simulink model "DynamicModel"  (R2021a)
settings: Solver=VariableStepAuto  StartTime=0.0  StopTime=10.0  RelTol=1e-3
libraries: pid_lib x2, simulink x1
settings Model: Creator=admin  LastModifiedBy=admin

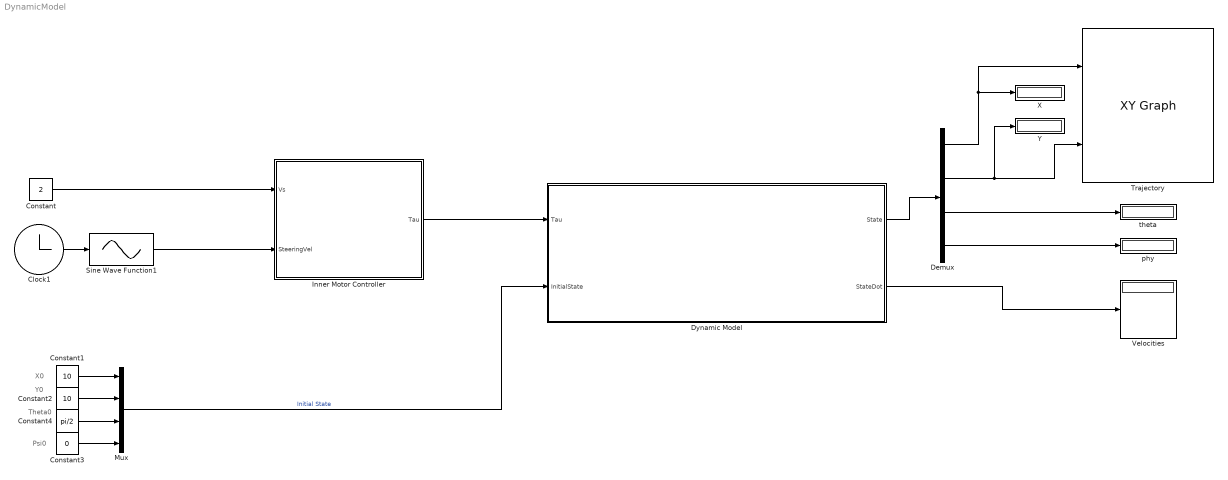
== system DynamicModel ==
  note: Y0
  note: X0
  note: Theta0
  note: Psi0
  Clock1 : Clock
  Constant : Constant  Value=2
  Constant1 : Constant  Value=10  SampleTime=0.001
  Constant2 : Constant  Value=10  SampleTime=0.001
  Constant3 : Constant  Value=0  SampleTime=0.001
  Constant4 : Constant  Value=pi/2  SampleTime=0.001
  Demux : Demux
  Dynamic Model : Subsystem
  Inner Motor Controller : Subsystem
  Mux : Mux
  Sine Wave Function1 : Sin  TimeSource=Use external signal  Amplitude=pi/4  Frequency=pi/2  SampleTime=0
  Trajectory : simulink/Sinks/XY Graph  xmin=-30  xmax=30  ymin=-30  ymax=30  st=0.001
  Velocities : Display
  X : Display
  Y : Display
  phy : Display
  theta : Display
  wires:
  Constant1/1 -> Mux/1
  Constant2/1 -> Mux/2
  Demux/3 -> theta/1
  Clock1/1 -> Sine Wave Function1/1
  Demux/2 -> Y/1, Trajectory/2
  Constant/1 -> Inner Motor Controller/1(Vs)
  Sine Wave Function1/1 -> Inner Motor Controller/2(SteeringVel)
  Constant4/1 -> Mux/3
  Demux/4 -> phy/1
  Demux/1 -> X/1, Trajectory/1
  Constant3/1 -> Mux/4
  Mux/1 -> Dynamic Model/2(InitialState)  "Initial State"
  Dynamic Model/2(StateDot) -> Velocities/1
  Dynamic Model/1(State) -> Demux/1
  Inner Motor Controller/1(Tau) -> Dynamic Model/1(Tau)

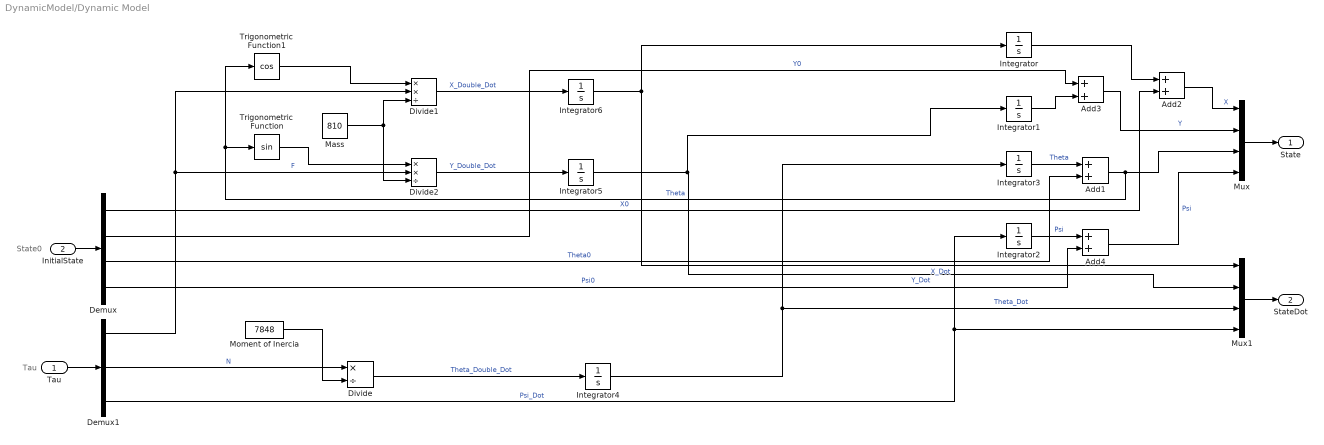
== system DynamicModel/Dynamic Model ==
  note: Tau
  note: State0
  Tau : Inport
  InitialState : Inport  Port=2
  Add{1..4} (4 alike) : Sum
  Demux : Demux
  Demux1 : Demux  Outputs=3
  Divide : Product  Inputs=*/
  Divide1 : Product  Inputs=**/
  Divide2 : Product  Inputs=**/
  Integrator{,1..6} (7 alike) : Integrator
  Mass : Constant  Value=810
  Moment of Inercia : Constant  Value=7848
  Mux : Mux
  Mux1 : Mux
  Trigonometric Function : Trigonometry
  Trigonometric Function1 : Trigonometry  Operator=cos
  State : Outport
  StateDot : Outport  Port=2
  wires:
  Mux/1 -> State/1
  Mux1/1 -> StateDot/1
  Demux1/3 -> Integrator2/1, Mux1/4  "Psi_Dot"
  Add4/1 -> Mux/4  "Psi"
  Add1/1 -> Trigonometric Function/1, Trigonometric Function1/1, Mux/3  "Theta"
  Integrator/1 -> Add2/1
  InitialState/1 -> Demux/1
  Add2/1 -> Mux/1  "X"
  Integrator1/1 -> Add3/2
  Add3/1 -> Mux/2  "Y"
  Tau/1 -> Demux1/1
  Demux/2 -> Add3/1  "Y0"
  Demux/1 -> Add2/2  "X0"
  Integrator3/1 -> Add1/1  "Theta"
  Demux/3 -> Add1/2  "Theta0"
  Integrator2/1 -> Add4/1  "Psi"
  Demux/4 -> Add4/2  "Psi0"
  Moment of Inercia/1 -> Divide/2
  Divide/1 -> Integrator4/1  "Theta_Double_Dot"
  Integrator4/1 -> Integrator3/1, Mux1/3  "Theta_Dot"
  Divide1/1 -> Integrator6/1  "X_Double_Dot"
  Divide2/1 -> Integrator5/1  "Y_Double_Dot"
  Demux1/2 -> Divide/1  "N"
  Trigonometric Function1/1 -> Divide1/1
  Trigonometric Function/1 -> Divide2/1
  Mass/1 -> Divide2/3, Divide1/3
  Demux1/1 -> Divide2/2, Divide1/2  "F"
  Integrator5/1 -> Integrator1/1, Mux1/2  "Y_Dot"
  Integrator6/1 -> Integrator/1, Mux1/1  "X_Dot"

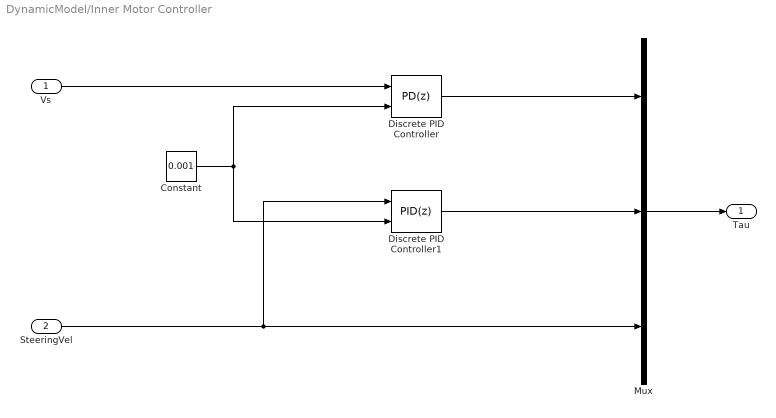
== system DynamicModel/Inner Motor Controller ==
  Vs : Inport
  SteeringVel : Inport  Port=2
  Constant : Constant  Value=0.001
  Discrete PID Controller : pid_lib/PID Controller  Controller=PD  Form=Parallel  TimeDomain=Discrete-time  UseExternalTs=on  SampleTime=-1  IntegratorMethod=Forward Euler  FilterMethod=Forward Euler  ControllerParametersSource=internal  P=1  I=1  D=0  UseFilter=on  N=100  TunerSelectOption=Transfer Function Based (PID Tuner App)  InitialConditionSource=internal  InitialConditionForIntegrator=0  InitialConditionForFilter=0  DifferentiatorICPrevScaledInput=0  ExternalReset=none  TrackingMode=off  Kt=1  LimitOutput=off  SatLimitsSource=internal  UpperSaturationLimit=inf  LowerSaturationLimit=-inf  LinearizeAsGain=off  AntiWindupMode=none  Kb=1  POutMin=[]  POutMax=[]  IOutMin=[]  IOutMax=[]  DOutMin=[]  DOutMax=[]  NOutMin=[]  NOutMax=[]  SumOutMin=[]  SumOutMax=[]  SaturationOutMin=[]  SaturationOutMax=[]  PParamMin=[]  PParamMax=[]  IParamMin=[]  IParamMax=[]  DParamMin=[]  DParamMax=[]  NParamMin=[]  NParamMax=[]  KbParamMin=[]  KbParamMax=[]  KtParamMin=[]  KtParamMax=[]  KbOutMin=[]  KbOutMax=[]  KtOutMin=[]  KtOutMax=[]  IntegratorOutMin=[]  IntegratorOutMax=[]  FilterOutMin=[]  FilterOutMax=[]  SumI1OutMin=[]  SumI1OutMax=[]  SumI2OutMin=[]  SumI2OutMax=[]  SumI3OutMin=[]  SumI3OutMax=[]  SumI4OutMin=[]  SumI4OutMax=[]  SumDOutMin=[]  SumDOutMax=[]  DifferentiatorOutMin=[]  DifferentiatorOutMax=[]  FilterDiffOutCoefMin=[]  FilterDiffOutCoefMax=[]  ReciprocalOutMin=[]  ReciprocalOutMax=[]  SumDenOutMin=[]  SumDenOutMax=[]  SumNumOutMin=[]  SumNumOutMax=[]  DivideOutMin=[]  DivideOutMax=[]  UdiffTsProdOutMin=[]  UdiffTsProdOutMax=[]  NTsProdOutMin=[]  NTsProdOutMax=[]  UintegralTsProdOutMin=[]  UintegralTsProdOutMax=[]  UngainTsProdOutMin=[]  UngainTsProdOutMax=[]  IntegratorContinuousStateAttributes=''  IntegratorStateMustResolveToSignalObject=off  IntegratorRTWStateStorageClass=Auto  FilterContinuousStateAttributes=''  FilterStateMustResolveToSignalObject=off  FilterRTWStateStorageClass=Auto  ParallelPVariant=InternalParameters  IdealPVariant=Disabled  IVariant=Disabled  DVariant=InternalParameters  IntegratorVariant=Disabled  SatVariant=Disabled  AWVariant=Disabled  PCopyVariant=Disabled  TRVariant=Disabled  FdbkBlocksVariant=Forward  IdealPFdbkVariant=Disabled  SatFdbkVariant=Disabled  DerivativeFilterVariant=ForwardEulerFilter  NVariant=InternalParameters  NCopyVariant=Disabled  FilterICVariant=InternalICsFilter  IntegratorICVariant=Disabled  ExternalResetVariant=Disabled  TRSumVariant=Passthrough  SumFdbkVariant=Disabled  SumVariant=Sum_PD  TsampFilterVariant=ExternalTs  TsampNgainVariant=ExternalTs  TsampIntegralVariant=Disabled  ExternalSaturationOutDataTypeStr=Inherit: Same as second input
  Discrete PID Controller1 : pid_lib/PID Controller  Controller=PID  Form=Parallel  TimeDomain=Discrete-time  UseExternalTs=on  SampleTime=-1  IntegratorMethod=Forward Euler  FilterMethod=Forward Euler  ControllerParametersSource=internal  P=1  I=1  D=0  UseFilter=on  N=100  TunerSelectOption=Transfer Function Based (PID Tuner App)  InitialConditionSource=internal  InitialConditionForIntegrator=0  InitialConditionForFilter=0  DifferentiatorICPrevScaledInput=0  ExternalReset=none  TrackingMode=off  Kt=1  LimitOutput=off  SatLimitsSource=internal  UpperSaturationLimit=inf  LowerSaturationLimit=-inf  LinearizeAsGain=off  AntiWindupMode=none  Kb=1  POutMin=[]  POutMax=[]  IOutMin=[]  IOutMax=[]  DOutMin=[]  DOutMax=[]  NOutMin=[]  NOutMax=[]  SumOutMin=[]  SumOutMax=[]  SaturationOutMin=[]  SaturationOutMax=[]  PParamMin=[]  PParamMax=[]  IParamMin=[]  IParamMax=[]  DParamMin=[]  DParamMax=[]  NParamMin=[]  NParamMax=[]  KbParamMin=[]  KbParamMax=[]  KtParamMin=[]  KtParamMax=[]  KbOutMin=[]  KbOutMax=[]  KtOutMin=[]  KtOutMax=[]  IntegratorOutMin=[]  IntegratorOutMax=[]  FilterOutMin=[]  FilterOutMax=[]  SumI1OutMin=[]  SumI1OutMax=[]  SumI2OutMin=[]  SumI2OutMax=[]  SumI3OutMin=[]  SumI3OutMax=[]  SumI4OutMin=[]  SumI4OutMax=[]  SumDOutMin=[]  SumDOutMax=[]  DifferentiatorOutMin=[]  DifferentiatorOutMax=[]  FilterDiffOutCoefMin=[]  FilterDiffOutCoefMax=[]  ReciprocalOutMin=[]  ReciprocalOutMax=[]  SumDenOutMin=[]  SumDenOutMax=[]  SumNumOutMin=[]  SumNumOutMax=[]  DivideOutMin=[]  DivideOutMax=[]  UdiffTsProdOutMin=[]  UdiffTsProdOutMax=[]  NTsProdOutMin=[]  NTsProdOutMax=[]  UintegralTsProdOutMin=[]  UintegralTsProdOutMax=[]  UngainTsProdOutMin=[]  UngainTsProdOutMax=[]  IntegratorContinuousStateAttributes=''  IntegratorStateMustResolveToSignalObject=off  IntegratorRTWStateStorageClass=Auto  FilterContinuousStateAttributes=''  FilterStateMustResolveToSignalObject=off  FilterRTWStateStorageClass=Auto  ParallelPVariant=InternalParameters  IdealPVariant=Disabled  IVariant=InternalParameters  DVariant=InternalParameters  IntegratorVariant=Discrete  SatVariant=Disabled  AWVariant=Passthrough  PCopyVariant=Disabled  TRVariant=Disabled  FdbkBlocksVariant=Forward  IdealPFdbkVariant=Disabled  SatFdbkVariant=Disabled  DerivativeFilterVariant=ForwardEulerFilter  NVariant=InternalParameters  NCopyVariant=Disabled  FilterICVariant=InternalICsFilter  IntegratorICVariant=InternalICs  ExternalResetVariant=Disabled  TRSumVariant=Passthrough  SumFdbkVariant=Disabled  SumVariant=Sum_PID  TsampFilterVariant=ExternalTs  TsampNgainVariant=ExternalTs  TsampIntegralVariant=ExternalTs  ExternalSaturationOutDataTypeStr=Inherit: Same as second input
  Mux : Mux  Inputs=3
  Tau : Outport
  wires:
  Mux/1 -> Tau/1
  SteeringVel/1 -> Discrete PID Controller1/1, Mux/3
  Constant/1 -> Discrete PID Controller/2, Discrete PID Controller1/2
  Vs/1 -> Discrete PID Controller/1
  Discrete PID Controller/1 -> Mux/1
  Discrete PID Controller1/1 -> Mux/2
